simulink library "Springs_Interconnected"  (R2020a)
settings: Solver=VariableStepAuto  StartTime=0.0  StopTime=10.0  RelTol=1e-3
libraries: sm_car_lib x3
Description:
  | Component of Simscape Vehicle Templates Library
  | 
  | Copyright 2018-2020 The MathWorks, Inc.
settings Model: Creator=smiller  LastModifiedBy=smiller
settings DataIOCC: ReturnWorkspaceOutputs=off
settings DebuggingCC: ArithmeticOperatorsInVariantConditions=warning
settings SFSimCC: CustomCodeUndefinedFunction=UseInterfaceOnly

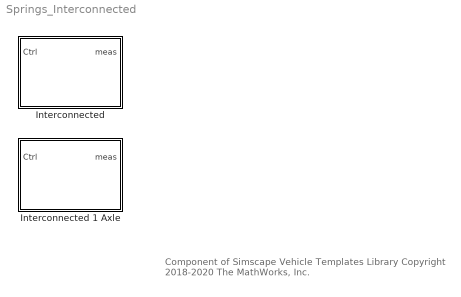
== system Springs_Interconnected ==
  note: Component of Simscape Vehicle Templates Library
      | Copyright 2018-2020 The MathWorks, Inc.
  Interconnected : Subsystem  VariantControl=Interconnected  mask(Interconnected Springs){InitTriggerDropdown=0}
      mask prompts: InitTriggerDropdown "Initialization Trigger Dropdown"
      mask help: Springs with connection across left and right sides.
      mask init:
      | curblk = gcb;
      | 
      | % Trigger Mask Initialization for 
      | % variant subsystems below this level
      | sm_car_lib_maskInitTrigger(curblk);
      mask TypeOptions InitTriggerDropdown: 0 | 1
  Interconnected 1 Axle : Subsystem  VariantControl=Interconnected  mask(Interconnected Springs){InitTriggerDropdown=0}
      mask prompts: InitTriggerDropdown "Initialization Trigger Dropdown"
      mask help: Springs with connection across left and right sides.
      mask init:
      | curblk = gcb;
      | 
      | % Trigger Mask Initialization for 
      | % variant subsystems below this level
      | sm_car_lib_maskInitTrigger(curblk);
      mask TypeOptions InitTriggerDropdown: 0 | 1

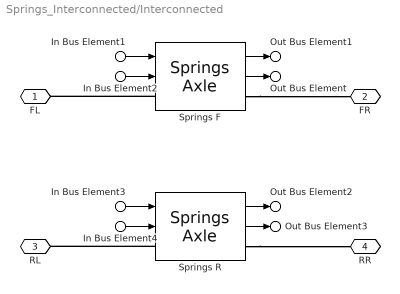
== system Springs_Interconnected/Interconnected ==
  In Bus Element1 : Inport  PortName=Ctrl  Element=FL
  In Bus Element2 : Inport  PortName=Ctrl  Element=FR
  In Bus Element3 : Inport  PortName=Ctrl  Element=RL
  In Bus Element4 : Inport  PortName=Ctrl  Element=RR
  Springs F : sm_car_lib/Springs Dampers/Springs Axle  VariantControl=Variant1  Spring=Spring.Front  VariantLabel=Spring.Front.class.Value  InitTriggerDropdown=0
  Springs R : sm_car_lib/Springs Dampers/Springs Axle  VariantControl=Variant1  Spring=Spring.Rear  VariantLabel=Spring.Rear.class.Value  InitTriggerDropdown=0
  FL : PMIOPort  Side=Left
  FR : PMIOPort  Port=2  Side=Right
  RL : PMIOPort  Port=3  Side=Left
  RR : PMIOPort  Port=4  Side=Right
  Out Bus Element : Outport  VectorParamsAs1DForOutWhenUnconnected=off  PortName=meas  Element=FL
  Out Bus Element1 : Outport  VectorParamsAs1DForOutWhenUnconnected=off  PortName=meas  Element=FR
  Out Bus Element2 : Outport  VectorParamsAs1DForOutWhenUnconnected=off  PortName=meas  Element=RL
  Out Bus Element3 : Outport  VectorParamsAs1DForOutWhenUnconnected=off  PortName=meas  Element=RR
  wires:
  Springs F/2 -> Out Bus Element/1
  Springs F/1 -> Out Bus Element1/1
  In Bus Element2/1 -> Springs F/2
  In Bus Element1/1 -> Springs F/1
  Springs R/2 -> Out Bus Element3/1
  Springs R/1 -> Out Bus Element2/1
  In Bus Element4/1 -> Springs R/2
  In Bus Element3/1 -> Springs R/1
  connections:
  Springs F/RConn1 -- FR/RConn1
  Springs F/LConn1 -- FL/RConn1
  Springs R/LConn1 -- RL/RConn1
  Springs R/RConn1 -- RR/RConn1

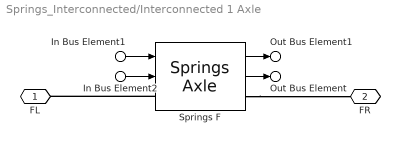
== system Springs_Interconnected/Interconnected 1 Axle ==
  In Bus Element1 : Inport  PortName=Ctrl  Element=FL
  In Bus Element2 : Inport  PortName=Ctrl  Element=FR
  Springs F : sm_car_lib/Springs Dampers/Springs Axle  VariantControl=Variant1  Spring=Spring.Front  VariantLabel=Spring.Front.class.Value  InitTriggerDropdown=0
  FL : PMIOPort  Side=Left
  FR : PMIOPort  Port=2  Side=Right
  Out Bus Element : Outport  VectorParamsAs1DForOutWhenUnconnected=off  PortName=meas  Element=FL
  Out Bus Element1 : Outport  VectorParamsAs1DForOutWhenUnconnected=off  PortName=meas  Element=FR
  wires:
  In Bus Element1/1 -> Springs F/1
  In Bus Element2/1 -> Springs F/2
  Springs F/1 -> Out Bus Element1/1
  Springs F/2 -> Out Bus Element/1
  connections:
  Springs F/LConn1 -- FL/RConn1
  Springs F/RConn1 -- FR/RConn1
